simulink model "surge_model"  (R2018a)
settings: Solver=ode45  StartTime=0.0  StopTime=tstop  RelTol=1e-3  EnableMultiTasking=on
values from neighbouring files (symbols this model uses):
  d_1 = 0    [run_task_1_8_new.m]
  d_2 = 1.0375    [run_task_1_8_new.m]
  m_u = 5500    [run_task_1_8_new.m]
  nc = 7.3    [run_task_1_4.m]    (also in run_task_1_6.m = nc_arr(i))
  tsamp = 10    [run_2.m]    (also in run_task_1_4.m; run_task_1_6.m; run_task_1_8_new.m)
  v0 = [6.63 0]'    [run_2.m]    (also in run_task_1_4.m; run_task_1_6.m = [0.001 0]'; run_task_1_8_new.m = [3 0]')
settings Model: Creator=ONL  LastModifiedBy=sondr
settings DataIOCC: LimitDataPoints=on  SaveFormat=Array
settings OptimizationCC: LifeSpan=inf
settings DebuggingCC: SFUnexpectedBacktrackingDiag=warning  SFNoUnconditionalDefaultTransitionDiag=warning  SFExecutionAtInitializationDiag=none
settings HardwareCC: ProdBitPerPointer=32  ProdBitPerSizeT=32  ProdBitPerPtrDiffT=32  ProdLargestAtomicFloat=None  ProdIntDivRoundTo=Undefined  ProdEndianess=Unspecified  ProdWordSize=32  ProdHWDeviceType=32-bit Generic
settings ModelReferenceCC: PropagateSignalLabelsOutOfModel=off
settings CodeAppCC: StateflowObjectComments=on
settings GRTTargetCC: TargetLangStandard=C89/C90 (ANSI)  GeneratePreprocessorConditionals=Disable all
settings ConfigComp: CovMetricSettings=dw  CovHtmlReporting=on  CovSaveCumulativeToWorkspaceVar=on  CovSaveSingleToWorkspaceVar=on  CovExternalEMLEnable=off

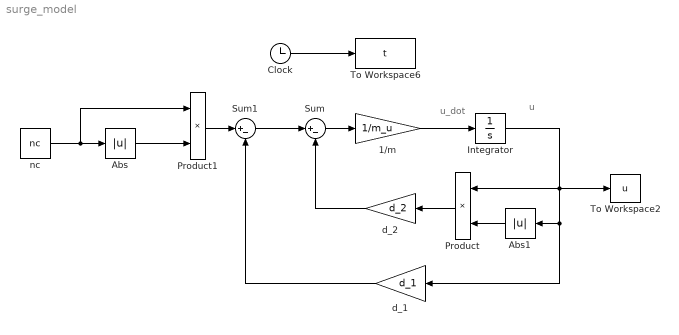
== system surge_model ==
  note: u
  note: u_dot
  1/m : Gain  Gain=1/m_u
  Abs : Abs
  Abs1 : Abs
  Clock : Clock
  Integrator : Integrator  InitialCondition=v0(1)
  Product : Product
  Product1 : Product
  Sum : Sum  Inputs=|+-
  Sum1 : Sum  Inputs=|+-
  To Workspace2 : ToWorkspace  VariableName=u  SampleTime=tsamp
  To Workspace6 : ToWorkspace  VariableName=t  SampleTime=tsamp
  d_1 : Gain  Gain=d_1
  d_2 : Gain  Gain=d_2
  nc : Constant  Value=nc
  wires:
  Clock/1 -> To Workspace6/1
  Integrator/1 -> To Workspace2/1, Product/1, d_1/1, Abs1/1
  nc/1 -> Product1/1, Abs/1
  Abs/1 -> Product1/2
  1/m/1 -> Integrator/1
  Sum/1 -> 1/m/1
  Sum1/1 -> Sum/1
  Product/1 -> d_2/1
  Abs1/1 -> Product/2
  Product1/1 -> Sum1/1
  d_2/1 -> Sum/2
  d_1/1 -> Sum1/2
